simulink model "ACCSystem"  (R2015a)
settings: Solver=FixedStepDiscrete  StartTime=0.0  StopTime=10  FixedStep=0.1  RelTol=1e-3
settings Model: Creator=Gugu  LastModifiedBy=Gugu
settings OptimizationCC: OptimizeModelRefInitCode=on  LifeSpan=1
settings HardwareCC: ProdLargestAtomicInteger=Long  ProdLargestAtomicFloat=Double  ProdEndianess=LittleEndian  ProdHWDeviceType=ARM Compatible->ARM Cortex
settings RTWCC: SystemTargetFile=ert.tlc  GenCodeOnly=on  TemplateMakefile=ert_default_tmf  Description=Embedded Coder  GenerateReport=on  IncludeHyperlinkInReport=on  LaunchReport=on  GenerateTraceInfo=on  GenerateTraceReport=on  GenerateTraceReportSl=on  GenerateTraceReportSf=on  GenerateTraceReportEml=on
settings CodeAppCC: IgnoreCustomStorageClasses=off
settings ERTTargetCC: ParMdlRefBuildCompliant=on  CompOptLevelCompliant=on  ConcurrentExecutionCompliant=on  ERTFirstTimeCompliant=on  MultiInstanceERTCode=on  CodeInterfacePackaging=Reusable function  SupportContinuousTime=off  SupportVariableSizeSignals=off  ModelStepFunctionPrototypeControlCompliant=on  CPPClassGenCompliant=on  InlinedParameterPlacement=Hierarchical  ERTCustomFileTemplate=example_file_process.tlc  ERTFilePackagingFormat=Compact

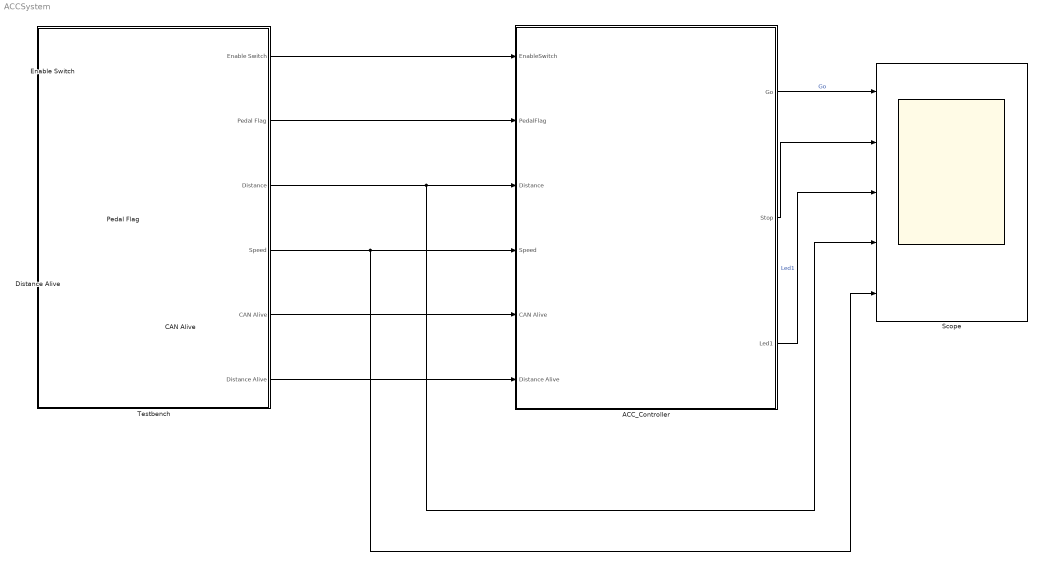
== system ACCSystem ==
  ACC_Controller : Subsystem
  CAN Alive : Subsystem  DialogController=hmiCreateDDGDialog  IsWebBlock=on  mask(MathWorksWebBlock){webBlockId=7722e2ce-702b-4f9e-8c54-58cd33225e31, webBlockType=toggleswitch, ShowInLibBrowser=on, ShowInitialText=on, HMISrcModelName=ACCSystem}
      mask prompts: webBlockId "WebBlock Id"; webBlockType "WebBlock Type"; HMISrcModelName "Source Model"
      mask Help: helpview([docroot '/mapfiles/simulink.map'], 'hmi_toggle_switch')
      mask Display:
      | if strcmp(get_param(bdroot(gcb),'BlockDiagramType'), 'library')
      |     image([(matlabroot) '/toolbox/simulink/hmi/icons/ToggleSwitch.png']);
      | end
  Distance Alive : Subsystem  DialogController=hmiCreateDDGDialog  IsWebBlock=on  mask(MathWorksWebBlock){webBlockId=6b0d6acb-485d-404e-b399-357eb8b03551, webBlockType=toggleswitch, ShowInLibBrowser=on, ShowInitialText=on, HMISrcModelName=ACCSystem}
      mask prompts: webBlockId "WebBlock Id"; webBlockType "WebBlock Type"; HMISrcModelName "Source Model"
      mask Help: helpview([docroot '/mapfiles/simulink.map'], 'hmi_toggle_switch')
      mask Display:
      | if strcmp(get_param(bdroot(gcb),'BlockDiagramType'), 'library')
      |     image([(matlabroot) '/toolbox/simulink/hmi/icons/ToggleSwitch.png']);
      | end
  Enable Switch : Subsystem  DialogController=hmiCreateDDGDialog  IsWebBlock=on  mask(MathWorksWebBlock){webBlockId=ee934517-a77b-44af-a230-e3552fc11bb6, webBlockType=discreteknob, ShowInLibBrowser=on, ShowInitialText=on, HMISrcModelName=ACCSystem}
      mask prompts: webBlockId "WebBlock Id"; webBlockType "WebBlock Type"; HMISrcModelName "Source Model"
      mask Help: helpview([docroot '/mapfiles/simulink.map'], 'hmi_rotary_switch')
      mask Display:
      | model = bdroot(gcb);
      | if strcmp(get_param(model,'BlockDiagramType'), 'library')
      |     image([(matlabroot) '/toolbox/simulink/hmi/icons/DiscreteKnob.png']);
      | end
  Pedal Flag : Subsystem  DialogController=hmiCreateDDGDialog  IsWebBlock=on  mask(MathWorksWebBlock){webBlockId=53fae0d6-1fc1-4d6f-838a-91792d26ca06, webBlockType=toggleswitch, ShowInLibBrowser=on, ShowInitialText=on, HMISrcModelName=ACCSystem}
      mask prompts: webBlockId "WebBlock Id"; webBlockType "WebBlock Type"; HMISrcModelName "Source Model"
      mask Help: helpview([docroot '/mapfiles/simulink.map'], 'hmi_toggle_switch')
      mask Display:
      | if strcmp(get_param(bdroot(gcb),'BlockDiagramType'), 'library')
      |     image([(matlabroot) '/toolbox/simulink/hmi/icons/ToggleSwitch.png']);
      | end
  Scope : Scope  NumInputPorts=5
      settings: YMin=86~76~-5~-5~-5  YMax=91~86.5~5~5~5
  Testbench : Subsystem
  wires:
  Testbench/1(Enable Switch) -> ACC_Controller/1(EnableSwitch)
  Testbench/2(Pedal Flag) -> ACC_Controller/2(PedalFlag)
  Testbench/3(Distance) -> Scope/4, ACC_Controller/3(Distance)
  Testbench/4(Speed) -> ACC_Controller/4(Speed), Scope/5
  ACC_Controller/1(Go) -> Scope/1  "Go"
  ACC_Controller/2(Stop) -> Scope/2
  Testbench/5(CAN Alive) -> ACC_Controller/5(CAN Alive)
  Testbench/6(Distance Alive) -> ACC_Controller/6(Distance Alive)
  ACC_Controller/3(Led1) -> Scope/3  "Led1"

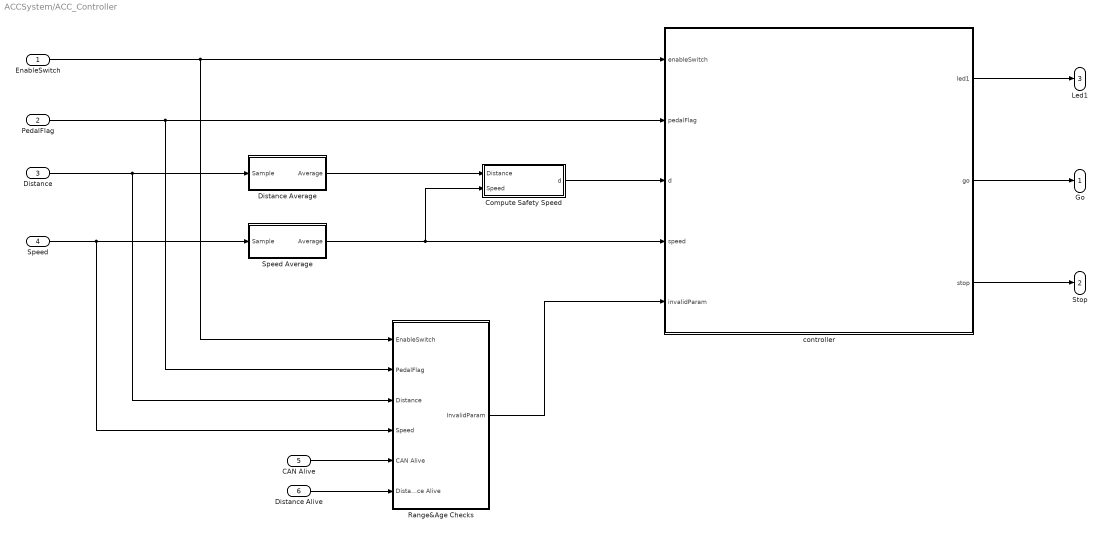
== system ACCSystem/ACC_Controller ==
  EnableSwitch : Inport
  PedalFlag : Inport  Port=2
  Distance : Inport  Port=3
  Speed : Inport  Port=4  OutDataTypeStr=double
  CAN Alive : Inport  Port=5  OutDataTypeStr=uint8
  Distance Alive : Inport  Port=6  OutDataTypeStr=uint8
  Compute Safety Speed : Subsystem
  Distance Average : Subsystem
  Range&Age Checks : Subsystem
  Speed Average : Subsystem
  controller : Stateflow chart  TreatAsAtomicUnit=on
  Go : Outport
  Stop : Outport  Port=2
  Led1 : Outport  Port=3
  wires:
  controller/1(led1) -> Led1/1
  controller/2(go) -> Go/1
  controller/3(stop) -> Stop/1
  EnableSwitch/1 -> Range&Age Checks/1(EnableSwitch), controller/1(enableSwitch)
  PedalFlag/1 -> controller/2(pedalFlag), Range&Age Checks/2(PedalFlag)
  Speed Average/1(Average) -> Compute Safety Speed/2(Speed), controller/4(speed)
  Distance/1 -> Distance Average/1(Sample), Range&Age Checks/3(Distance)
  Distance Average/1(Average) -> Compute Safety Speed/1(Distance)
  Compute Safety Speed/1(d) -> controller/3(d)
  Speed/1 -> Speed Average/1(Sample), Range&Age Checks/4(Speed)
  CAN Alive/1 -> Range&Age Checks/5(CAN Alive)
  Distance Alive/1 -> Range&Age Checks/6(Distance Alive)
  Range&Age Checks/1(InvalidParam) -> controller/5(invalidParam)

== system ACCSystem/CAN Alive ==

== system ACCSystem/Distance Alive ==

== system ACCSystem/Enable Switch ==

== system ACCSystem/Pedal Flag ==

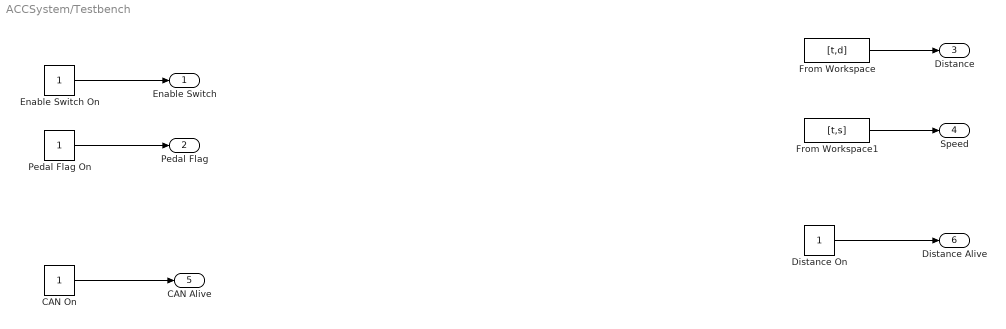
== system ACCSystem/Testbench ==
  CAN On : Constant  OutDataTypeStr=uint8
  Distance On : Constant  OutDataTypeStr=uint8
  Enable Switch On : Constant  OutDataTypeStr=uint8
  From Workspace : FromWorkspace  VariableName=[t,d]
  From Workspace1 : FromWorkspace  VariableName=[t,s]
  Pedal Flag On : Constant  OutDataTypeStr=uint8
  Enable Switch : Outport
  Pedal Flag : Outport  Port=2
  Distance : Outport  Port=3
  Speed : Outport  Port=4
  CAN Alive : Outport  Port=5
  Distance Alive : Outport  Port=6
  wires:
  Enable Switch On/1 -> Enable Switch/1
  Pedal Flag On/1 -> Pedal Flag/1
  From Workspace/1 -> Distance/1
  From Workspace1/1 -> Speed/1
  CAN On/1 -> CAN Alive/1
  Distance On/1 -> Distance Alive/1

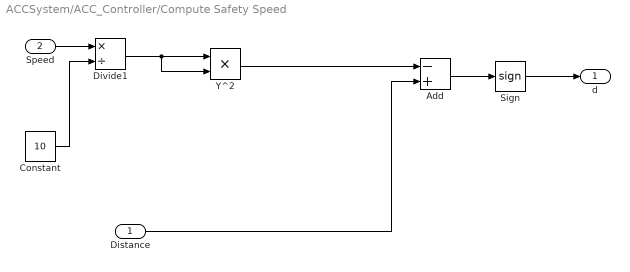
== system ACCSystem/ACC_Controller/Compute Safety Speed ==
  Distance : Inport  OutDataTypeStr=double
  Speed : Inport  Port=2  OutDataTypeStr=double
  Add : Sum  Inputs=-+
  Constant : Constant  Value=10  OutDataTypeStr=double
  Divide1 : Product  Inputs=*/
  Sign : Signum
  Y^2 : Product  OutDataTypeStr=double
  d : Outport  OutDataTypeStr=double
  wires:
  Constant/1 -> Divide1/2
  Speed/1 -> Divide1/1
  Divide1/1 -> Y^2/2, Y^2/1
  Distance/1 -> Add/2
  Add/1 -> Sign/1
  Y^2/1 -> Add/1
  Sign/1 -> d/1

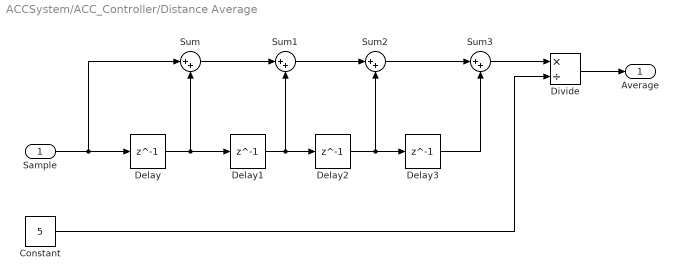
== system ACCSystem/ACC_Controller/Distance Average ==
  Sample : Inport
  Constant : Constant  Value=5  OutDataTypeStr=double
  Delay{,1..3} (4 alike) : Delay  DelayLength=1  InitialCondition=0
  Divide : Product  Inputs=*/
  Sum{,1..3} (4 alike) : Sum  Inputs=|++
  Average : Outport
  wires:
  Sample/1 -> Sum/1, Delay/1
  Delay/1 -> Sum/2, Delay1/1
  Delay1/1 -> Sum1/2, Delay2/1
  Delay2/1 -> Sum2/2, Delay3/1
  Sum/1 -> Sum1/1
  Sum1/1 -> Sum2/1
  Sum2/1 -> Sum3/1
  Delay3/1 -> Sum3/2
  Sum3/1 -> Divide/1
  Divide/1 -> Average/1
  Constant/1 -> Divide/2

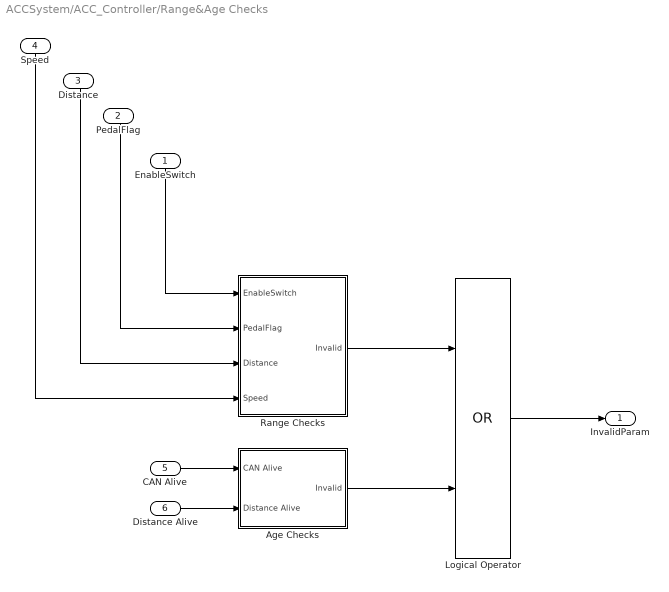
== system ACCSystem/ACC_Controller/Range&Age Checks ==
  EnableSwitch : Inport
  PedalFlag : Inport  Port=2
  Distance : Inport  Port=3
  Speed : Inport  Port=4
  CAN Alive : Inport  Port=5  OutDataTypeStr=uint8
  Distance Alive : Inport  Port=6  OutDataTypeStr=uint8
  Age Checks : Subsystem
  Logical Operator : Logic  Operator=OR  AllPortsSameDT=off  OutDataTypeStr=boolean
  Range Checks : Subsystem
  InvalidParam : Outport
  wires:
  Logical Operator/1 -> InvalidParam/1
  Range Checks/1(Invalid) -> Logical Operator/1
  Age Checks/1(Invalid) -> Logical Operator/2
  Distance Alive/1 -> Age Checks/2(Distance Alive)
  CAN Alive/1 -> Age Checks/1(CAN Alive)
  Speed/1 -> Range Checks/4(Speed)
  PedalFlag/1 -> Range Checks/2(PedalFlag)
  Distance/1 -> Range Checks/3(Distance)
  EnableSwitch/1 -> Range Checks/1(EnableSwitch)

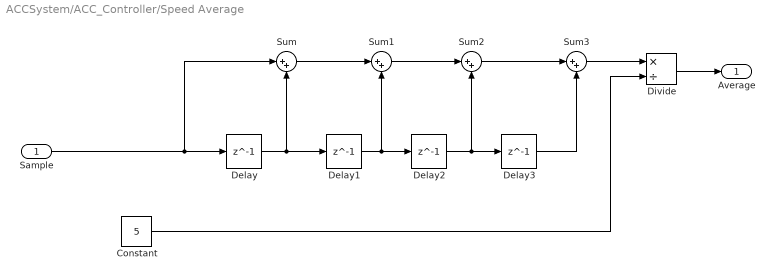
== system ACCSystem/ACC_Controller/Speed Average ==
  Sample : Inport  OutDataTypeStr=double
  Constant : Constant  Value=5  OutDataTypeStr=double
  Delay{,1..3} (4 alike) : Delay  DelayLength=1  InitialCondition=0
  Divide : Product  Inputs=*/
  Sum{,1..3} (4 alike) : Sum  Inputs=|++
  Average : Outport  OutDataTypeStr=double
  wires:
  Sample/1 -> Sum/1, Delay/1
  Delay/1 -> Sum/2, Delay1/1
  Delay1/1 -> Sum1/2, Delay2/1
  Delay2/1 -> Sum2/2, Delay3/1
  Sum/1 -> Sum1/1
  Sum1/1 -> Sum2/1
  Sum2/1 -> Sum3/1
  Delay3/1 -> Sum3/2
  Sum3/1 -> Divide/1
  Divide/1 -> Average/1
  Constant/1 -> Divide/2

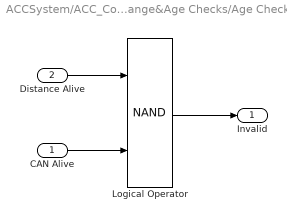
== system ACCSystem/ACC_Controller/Range&Age Checks/Age Checks ==
  CAN Alive : Inport
  Distance Alive : Inport  Port=2  OutDataTypeStr=uint8
  Logical Operator : Logic  Operator=NAND  AllPortsSameDT=off  OutDataTypeStr=boolean
  Invalid : Outport
  wires:
  Logical Operator/1 -> Invalid/1
  CAN Alive/1 -> Logical Operator/2
  Distance Alive/1 -> Logical Operator/1

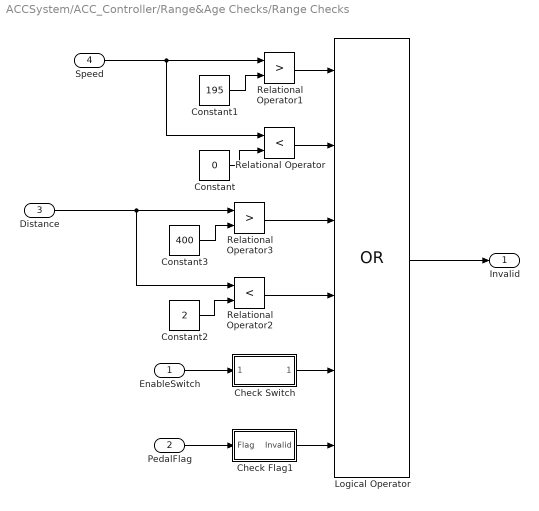
== system ACCSystem/ACC_Controller/Range&Age Checks/Range Checks ==
  EnableSwitch : Inport
  PedalFlag : Inport  Port=2
  Distance : Inport  Port=3
  Speed : Inport  Port=4  OutDataTypeStr=double
  Check Flag1 : Subsystem
  Check Switch : Subsystem
  Constant : Constant  Value=0  OutDataTypeStr=double
  Constant1 : Constant  Value=195  OutDataTypeStr=double
  Constant2 : Constant  Value=2  OutDataTypeStr=double
  Constant3 : Constant  Value=400  OutDataTypeStr=double
  Logical Operator : Logic  Operator=OR  Inputs=6  AllPortsSameDT=off  OutDataTypeStr=boolean
  Relational Operator : RelationalOperator  Operator=<  OutDataTypeStr=boolean
  Relational Operator1 : RelationalOperator  Operator=>  OutDataTypeStr=boolean
  Relational Operator2 : RelationalOperator  Operator=<  OutDataTypeStr=boolean
  Relational Operator3 : RelationalOperator  Operator=>  OutDataTypeStr=boolean
  Invalid : Outport
  wires:
  Speed/1 -> Relational Operator/1, Relational Operator1/1
  Constant/1 -> Relational Operator/2
  Constant1/1 -> Relational Operator1/2
  Distance/1 -> Relational Operator2/1, Relational Operator3/1
  Constant2/1 -> Relational Operator2/2
  Constant3/1 -> Relational Operator3/2
  Relational Operator/1 -> Logical Operator/2
  Relational Operator3/1 -> Logical Operator/3
  Relational Operator2/1 -> Logical Operator/4
  Relational Operator1/1 -> Logical Operator/1
  Logical Operator/1 -> Invalid/1
  PedalFlag/1 -> Check Flag1/1(Flag)
  EnableSwitch/1 -> Check Switch/1(Switch)
  Check Switch/1(Invalid) -> Logical Operator/5
  Check Flag1/1(Invalid) -> Logical Operator/6

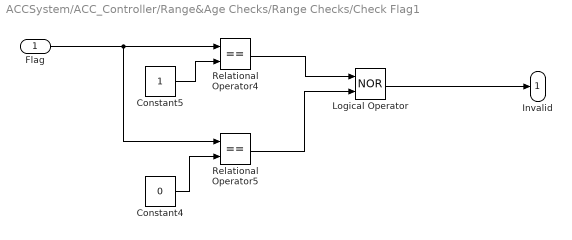
== system ACCSystem/ACC_Controller/Range&Age Checks/Range Checks/Check Flag1 ==
  Flag : Inport  OutDataTypeStr=uint8
  Constant4 : Constant  Value=0  OutDataTypeStr=uint8
  Constant5 : Constant  OutDataTypeStr=uint8
  Logical Operator : Logic  Operator=NOR  AllPortsSameDT=off  OutDataTypeStr=boolean
  Relational Operator4 : RelationalOperator  Operator===  OutDataTypeStr=boolean
  Relational Operator5 : RelationalOperator  Operator===  OutDataTypeStr=boolean
  Invalid : Outport
  wires:
  Relational Operator4/1 -> Logical Operator/1
  Constant4/1 -> Relational Operator5/2
  Constant5/1 -> Relational Operator4/2
  Relational Operator5/1 -> Logical Operator/2
  Flag/1 -> Relational Operator5/1, Relational Operator4/1
  Logical Operator/1 -> Invalid/1

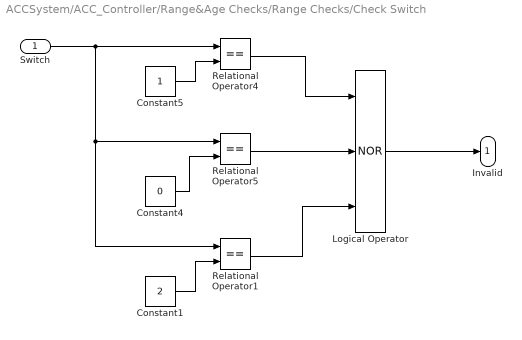
== system ACCSystem/ACC_Controller/Range&Age Checks/Range Checks/Check Switch ==
  Switch : Inport  OutDataTypeStr=uint8
  Constant1 : Constant  Value=2  OutDataTypeStr=uint8
  Constant4 : Constant  Value=0  OutDataTypeStr=uint8
  Constant5 : Constant  OutDataTypeStr=uint8
  Logical Operator : Logic  Operator=NOR  Inputs=3  AllPortsSameDT=off  OutDataTypeStr=boolean
  Relational Operator1 : RelationalOperator  Operator===  OutDataTypeStr=boolean
  Relational Operator4 : RelationalOperator  Operator===  OutDataTypeStr=boolean
  Relational Operator5 : RelationalOperator  Operator===  OutDataTypeStr=boolean
  Invalid : Outport
  wires:
  Relational Operator4/1 -> Logical Operator/1
  Constant4/1 -> Relational Operator5/2
  Constant5/1 -> Relational Operator4/2
  Relational Operator5/1 -> Logical Operator/2
  Switch/1 -> Relational Operator5/1, Relational Operator1/1, Relational Operator4/1
  Logical Operator/1 -> Invalid/1
  Constant1/1 -> Relational Operator1/2
  Relational Operator1/1 -> Logical Operator/3

== stateflow chart ACCSystem/ACC_Controller/controller ==
  state OFF_STATE
    en:
    led1=uint8(0)
  state ON_STATE
    ex:
    stop = uint8(0)
    go = uint8(0)
    state WAIT
    state INIT_ON
      en:
      led1=uint8(1)
      setSpeed = speed
    state IDLE_STATE
      en:
      go=uint8(0)
      stop=uint8(0)
    state WORKING_STATE
      state STOP_STATE
        en:
        go=uint8(0)
        stop= uint8(1)
      state GO_STATE
        en:
        go=uint8(1)
        stop=uint8(0)
      GO_STATE -> STOP_STATE : [d < 0 || speed > setSpeed]
      STOP_STATE -> GO_STATE : [d > 0 && speed < setSpeed]
    (default) -> WAIT
    WAIT -> INIT_ON : after(4, tick)
    INIT_ON -> IDLE_STATE
    IDLE_STATE -> IDLE_STATE [order 1] : [speed == 0]
    IDLE_STATE -> STOP_STATE [order 2] : [d < 0 || speed > setSpeed]
    IDLE_STATE -> GO_STATE [order 3] : [d > 0 && speed < setSpeed]
    WORKING_STATE -> IDLE_STATE : [speed == 0 || (d == 0 && speed <= setSpeed) || (d >= 0 && speed == setSpeed)]
  state OVERRIDDEN_STATE
    en:
    led1=uint8(2)
  OFF_STATE -> ON_STATE : [pedalFlag==0 && enableSwitch==1]
  (default) -> OFF_STATE
  OVERRIDDEN_STATE -> OFF_STATE [order 1] : [enableSwitch==0]
  ON_STATE -> OFF_STATE [order 1] : [enableSwitch==0]
  OVERRIDDEN_STATE -> ON_STATE [order 3] : [enableSwitch==2]
  OVERRIDDEN_STATE -> OVERRIDDEN_STATE [order 2] : [pedalFlag==1 || invalidParam == 1]
  ON_STATE -> OVERRIDDEN_STATE [order 2] : [pedalFlag==1 || invalidParam == 1]
  data: enableSwitch input uint8 size=1; led1 output uint8 size=1; pedalFlag input uint8 size=1; d input double size=1; speed input double size=1; go output uint8 size=1; stop output uint8 size=1; setSpeed local; invalidParam input boolean
